simulink model "gm_stream_adaptation_model"  (R2020b)
settings: Solver=FixedStepDiscrete  StartTime=0.0  StopTime=2  RelTol=1e-3
undefined symbols (not defined in the file or in its folder): frame
libraries: hdlmdlgenlib x16, hdlsllib x2, simulink x2, whdlio x1
settings Model: Creator=wardo  LastModifiedBy=wardo
settings DataIOCC: LimitDataPoints=on  SaveOutput=off  SaveTime=off
settings OptimizationCC: BlockReduction=off  ConditionallyExecuteInputs=off  DefaultParameterBehavior=Inlined  LifeSpan=inf
settings DebuggingCC: AlgebraicLoopMsg=error  InheritedTsInSrcMsg=none  SingleTaskRateTransMsg=error  AllowSymbolicDim=off  StrictBusMsg=ErrorOnBusTreatedAsVector  SFUnexpectedBacktrackingDiag=warning  SFNoUnconditionalDefaultTransitionDiag=warning  SFExecutionAtInitializationDiag=none  ArithmeticOperatorsInVariantConditions=warning
settings HardwareCC: ProdBitPerPointer=32  ProdBitPerSizeT=32  ProdBitPerPtrDiffT=32  ProdLargestAtomicFloat=None  ProdIntDivRoundTo=Undefined  ProdEndianess=Unspecified  ProdWordSize=32  ProdHWDeviceType=ASIC/FPGA->ASIC/FPGA  ProdEqTarget=off
settings SFSimCC: SimUseLocalCustomCode=off  CustomCodeUndefinedFunction=UseInterfaceOnly
settings RTWCC: RTWUseLocalCustomCode=off
settings CodeAppCC: StateflowObjectComments=on
settings GRTTargetCC: TargetLangStandard=C89/C90 (ANSI)
settings ConfigComp: CovScope=ReferencedModels  CovMetricSettings=dw  CovSaveCumulativeToWorkspaceVar=on  CovSaveSingleToWorkspaceVar=on  CovExternalEMLEnable=off  CovSFcnEnable=off

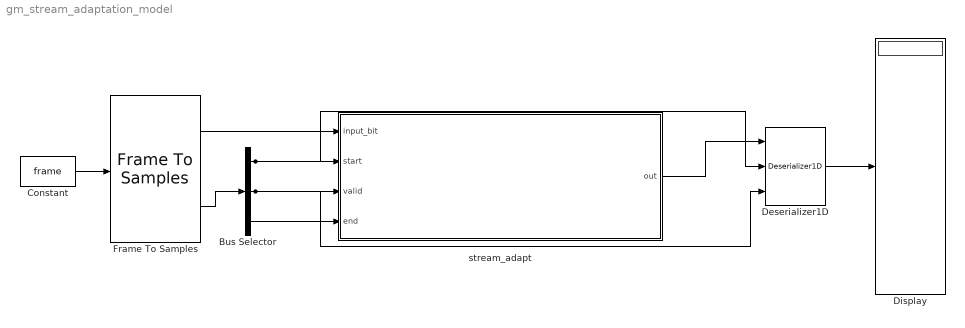
== system gm_stream_adaptation_model ==
  Bus Selector : BusSelector  OutputSignals=start,valid,end
  Constant : Constant  Value=frame  OutDataTypeStr=fixdt(1,16)  SampleTime=1
  Deserializer1D : hdlsllib/HDL Operations/Deserializer1D  Ratio=48408  IdleCycles=0  InitialCondition=0  startIn=on  validIn=on  validOut=off  inputDataDimensions=-1  inputSampleTime=-1  inputSignalType=auto
      settings: SourceProductBaseCode=SL
  Display : Display
  Frame To Samples : whdlio/Frame To Samples  InterSampleIdleCycles=0  InterFrameIdleCycles=0  OutputSize=1  InterleaveSamples=off
      settings: SourceProductBaseCode=LH
  stream_adapt : Subsystem
  wires:
  Deserializer1D/1 -> Display/1
  stream_adapt/1(out) -> Deserializer1D/1
  Bus Selector/3 -> stream_adapt/4(end)
  Bus Selector/2 -> stream_adapt/3(valid), Deserializer1D/3
  Bus Selector/1 -> stream_adapt/2(start), Deserializer1D/2
  Frame To Samples/2 -> Bus Selector/1
  Frame To Samples/1 -> stream_adapt/1(input_bit)
  Constant/1 -> Frame To Samples/1

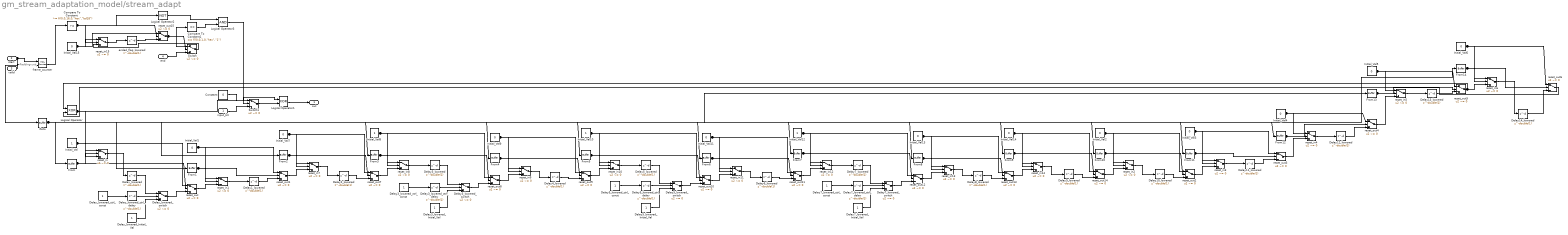
== system gm_stream_adaptation_model/stream_adapt ==
  note: Padding unit
  input_bit : Inport  OutDataTypeStr=fixdt(1, 16, 14)  PortDimensions=1  SampleTime=2.06577425218972e-05
  start : Inport  Port=2  OutDataTypeStr=boolean  PortDimensions=1  SampleTime=2.06577425218972e-05
  valid : Inport  Port=3  OutDataTypeStr=boolean  PortDimensions=1  SampleTime=2.06577425218972e-05
  end : Inport  Port=4  OutDataTypeStr=boolean  PortDimensions=1  SampleTime=2.06577425218972e-05
  Compare To Constant : simulink/Logic and Bit Operations/Compare To Constant  relop=>=  const="fi(0,0,16,0,\"hex\",\"bd18\")"  OutDataTypeStr=boolean
  Compare To Constant1 : simulink/Logic and Bit Operations/Compare To Constant  relop===  const="fi(0,0,1,0,\"hex\",\"1\")"  OutDataTypeStr=boolean
  Constant : Constant  Value=0  OutDataTypeStr=fixdt(0, 1, 1000)  SampleTime=2.06577425218972e-05
  Delay10_lowered : Delay  DelayLength=double(1)  InitialCondition=0  SampleTime=2.06577425218972e-05
  Delay11_lowered : Delay  DelayLength=double(1)  InitialCondition=0  SampleTime=2.06577425218972e-05
  Delay12_lowered : Delay  DelayLength=double(1)  InitialCondition=0  SampleTime=2.06577425218972e-05
  Delay13_lowered : Delay  DelayLength=double(1)  InitialCondition=0  SampleTime=2.06577425218972e-05
  Delay14_lowered : Delay  DelayLength=double(1)  InitialCondition=0  SampleTime=2.06577425218972e-05
  Delay1_lowered : Delay  DelayLength=double(1)  InitialCondition=0  SampleTime=2.06577425218972e-05
  Delay2_lowered : Delay  DelayLength=double(1)  InitialCondition=0  SampleTime=2.06577425218972e-05
  Delay3_lowered : Delay  DelayLength=double(1)  InitialCondition=0  SampleTime=2.06577425218972e-05
  Delay3_lowered_Initial_Val : Constant  OutDataTypeStr=boolean  SampleTime=2.06577425218972e-05
  Delay3_lowered_ctrl_const : Constant  OutDataTypeStr=boolean  SampleTime=2.06577425218972e-05
  Delay3_lowered_ctrl_delay : Delay  DelayLength=double(1)  InitialCondition=0  SampleTime=2.06577425218972e-05
  Delay3_lowered_switch : Switch  Criteria=u2 ~= 0  Threshold=double(0)  OutDataTypeStr=boolean  SampleTime=2.06577425218972e-05
  Delay4_lowered : Delay  DelayLength=double(1)  InitialCondition=0  SampleTime=2.06577425218972e-05
  Delay5_lowered : Delay  DelayLength=double(1)  InitialCondition=0  SampleTime=2.06577425218972e-05
  Delay5_lowered_Initial_Val : Constant  OutDataTypeStr=boolean  SampleTime=2.06577425218972e-05
  Delay5_lowered_ctrl_const : Constant  OutDataTypeStr=boolean  SampleTime=2.06577425218972e-05
  Delay5_lowered_ctrl_delay : Delay  DelayLength=double(1)  InitialCondition=0  SampleTime=2.06577425218972e-05
  Delay5_lowered_switch : Switch  Criteria=u2 ~= 0  Threshold=double(0)  OutDataTypeStr=boolean  SampleTime=2.06577425218972e-05
  Delay6_lowered : Delay  DelayLength=double(1)  InitialCondition=0  SampleTime=2.06577425218972e-05
  Delay7_lowered : Delay  DelayLength=double(1)  InitialCondition=0  SampleTime=2.06577425218972e-05
  Delay7_lowered_Initial_Val : Constant  OutDataTypeStr=boolean  SampleTime=2.06577425218972e-05
  Delay7_lowered_ctrl_const : Constant  OutDataTypeStr=boolean  SampleTime=2.06577425218972e-05
  Delay7_lowered_ctrl_delay : Delay  DelayLength=double(1)  InitialCondition=0  SampleTime=2.06577425218972e-05
  Delay7_lowered_switch : Switch  Criteria=u2 ~= 0  Threshold=double(0)  OutDataTypeStr=boolean  SampleTime=2.06577425218972e-05
  Delay8_lowered : Delay  DelayLength=double(1)  InitialCondition=0  SampleTime=2.06577425218972e-05
  Delay9_lowered : Delay  DelayLength=double(1)  InitialCondition=0  SampleTime=2.06577425218972e-05
  Delay_lowered : Delay  DelayLength=double(1)  InitialCondition=0  SampleTime=2.06577425218972e-05
  Delay_lowered_Initial_Val : Constant  OutDataTypeStr=boolean  SampleTime=2.06577425218972e-05
  Delay_lowered_ctrl_const : Constant  OutDataTypeStr=boolean  SampleTime=2.06577425218972e-05
  Delay_lowered_ctrl_delay : Delay  DelayLength=double(1)  InitialCondition=0  SampleTime=2.06577425218972e-05
  Delay_lowered_switch : Switch  Criteria=u2 ~= 0  Threshold=double(0)  OutDataTypeStr=boolean  SampleTime=2.06577425218972e-05
  From{,1..14} (15 alike) : hdlmdlgenlib/Buffer
      settings: SourceProductBaseCode=SL
  Goto : hdlmdlgenlib/Buffer
      settings: SourceProductBaseCode=SL
  Initial_Val{,8,10,12} (4 alike) : Constant  OutDataTypeStr=boolean  SampleTime=2.06577425218972e-05
  Initial_Val{1..7,9,11,13..15} (12 alike) : Constant  Value=0  OutDataTypeStr=boolean  SampleTime=2.06577425218972e-05
  Logical Operator : Logic  Operator=XOR  AllPortsSameDT=off  OutDataTypeStr=boolean  SampleTime=2.06577425218972e-05
  Logical Operator1 : Logic  Operator=XOR  AllPortsSameDT=off  OutDataTypeStr=boolean  SampleTime=2.06577425218972e-05
  Logical Operator2 : Logic  Operator=NOT  Inputs=1  AllPortsSameDT=off  OutDataTypeStr=boolean  SampleTime=2.06577425218972e-05
  Logical Operator3 : Logic  AllPortsSameDT=off  OutDataTypeStr=boolean  SampleTime=2.06577425218972e-05
  Switch : Switch  Criteria=u2 ~= 0  Threshold=double(0)  OutDataTypeStr=boolean  SampleTime=2.06577425218972e-05
  Switch1 : Switch  Criteria=u2 ~= 0  Threshold=double(0)  OutDataTypeStr=fixdt(1, 16, 14)  SampleTime=2.06577425218972e-05
  ended_flag_lowered : Delay  DelayLength=double(1)  InitialCondition=0  SampleTime=2.06577425218972e-05
  frame_counter : hdlsllib/Sources/HDL Counter  CountType=Count limited  CountInit=double(0)  CountStep=double(1)  CountMax=double(48408)  CountFromType=Initial value  CountFrom=double(0)  CountResetPort=on  CountLoadPort=off  CountEnbPort=on  CountDirPort=off  CountDataType=Unsigned  CountWordLen=16  CountFracLen=0  CountSampTime=2.06577425218972e-05
  reset_in{,1..15} (16 alike) : Switch  Criteria=u2 ~= 0  Threshold=double(0)  OutDataTypeStr=boolean  SampleTime=2.06577425218972e-05
  reset_out{,1..15} (16 alike) : Switch  Criteria=u2 ~= 0  Threshold=double(0)  OutDataTypeStr=boolean  SampleTime=2.06577425218972e-05
  out : Outport  VectorParamsAs1DForOutWhenUnconnected=off
  wires:
  input_bit/1 -> Switch1/3
  start/1 -> frame_counter/1, Goto/1
  valid/1 -> frame_counter/2
  end/1 -> Switch/3
  Compare To Constant/1 -> Logical Operator2/1, reset_out15/2, reset_in15/2
  Compare To Constant1/1 -> Logical Operator3/2
  Constant/1 -> Switch1/1
  reset_out/1 -> reset_in1/3
  reset_out1/1 -> reset_in7/3
  reset_out2/1 -> reset_in3/3
  reset_out3/1 -> reset_in4/3
  reset_out4/1 -> reset_in5/3
  reset_out5/1 -> Logical Operator/1, reset_in6/3
  reset_out6/1 -> Logical Operator/2
  reset_out7/1 -> reset_in8/3
  reset_out8/1 -> reset_in9/3
  reset_out9/1 -> reset_in10/3
  reset_out10/1 -> reset_in11/3
  reset_out11/1 -> reset_in12/3
  reset_out12/1 -> reset_in13/3
  reset_out13/1 -> reset_in14/3
  reset_out14/1 -> reset_in2/3
  From/1 -> reset_out/2, reset_in/2
  From1/1 -> reset_out1/2, reset_in1/2
  From10/1 -> reset_out2/2, reset_in2/2
  From11/1 -> reset_out3/2, reset_in3/2
  From12/1 -> reset_out4/2, reset_in4/2
  From13/1 -> reset_out5/2, reset_in5/2
  From14/1 -> reset_out6/2, reset_in6/2
  From2/1 -> reset_out7/2, reset_in7/2
  From3/1 -> reset_out8/2, reset_in8/2
  From4/1 -> reset_out9/2, reset_in9/2
  From5/1 -> reset_out10/2, reset_in10/2
  From6/1 -> reset_out11/2, reset_in11/2
  From7/1 -> reset_out12/2, reset_in12/2
  From8/1 -> reset_out13/2, reset_in13/2
  From9/1 -> reset_out14/2, reset_in14/2
  Logical Operator/1 -> Logical Operator1/1, reset_in/3
  Logical Operator1/1 -> out/1
  Logical Operator2/1 -> Logical Operator3/1
  Logical Operator3/1 -> Switch1/2
  Switch/1 -> reset_in15/3
  Switch1/1 -> Logical Operator1/2
  reset_out15/1 -> Switch/2, Switch/1, Compare To Constant1/1
  frame_counter/1 -> Compare To Constant/1
  Goto/1 -> From9/1, From8/1, From7/1, From6/1, From5/1, From4/1, From3/1, From2/1, From14/1, From13/1, From12/1, From11/1, From10/1, From1/1, From/1
  Initial_Val/1 -> reset_out/1, reset_in/1
  Delay_lowered_switch/1 -> reset_out/3
  reset_in/1 -> Delay_lowered/1
  Initial_Val1/1 -> reset_out1/1, reset_in1/1
  Delay1_lowered/1 -> reset_out1/3
  reset_in1/1 -> Delay1_lowered/1
  Initial_Val2/1 -> reset_out2/1, reset_in2/1
  Delay10_lowered/1 -> reset_out2/3
  reset_in2/1 -> Delay10_lowered/1
  Initial_Val3/1 -> reset_out3/1, reset_in3/1
  Delay11_lowered/1 -> reset_out3/3
  reset_in3/1 -> Delay11_lowered/1
  Initial_Val4/1 -> reset_out4/1, reset_in4/1
  Delay12_lowered/1 -> reset_out4/3
  reset_in4/1 -> Delay12_lowered/1
  Initial_Val5/1 -> reset_out5/1, reset_in5/1
  Delay13_lowered/1 -> reset_out5/3
  reset_in5/1 -> Delay13_lowered/1
  Initial_Val6/1 -> reset_out6/1, reset_in6/1
  Delay14_lowered/1 -> reset_out6/3
  reset_in6/1 -> Delay14_lowered/1
  Initial_Val7/1 -> reset_out7/1, reset_in7/1
  Delay2_lowered/1 -> reset_out7/3
  reset_in7/1 -> Delay2_lowered/1
  Initial_Val8/1 -> reset_out8/1, reset_in8/1
  Delay3_lowered_switch/1 -> reset_out8/3
  reset_in8/1 -> Delay3_lowered/1
  Initial_Val9/1 -> reset_out9/1, reset_in9/1
  Delay4_lowered/1 -> reset_out9/3
  reset_in9/1 -> Delay4_lowered/1
  Initial_Val10/1 -> reset_out10/1, reset_in10/1
  Delay5_lowered_switch/1 -> reset_out10/3
  reset_in10/1 -> Delay5_lowered/1
  Initial_Val11/1 -> reset_out11/1, reset_in11/1
  Delay6_lowered/1 -> reset_out11/3
  reset_in11/1 -> Delay6_lowered/1
  Initial_Val12/1 -> reset_out12/1, reset_in12/1
  Delay7_lowered_switch/1 -> reset_out12/3
  reset_in12/1 -> Delay7_lowered/1
  Initial_Val13/1 -> reset_out13/1, reset_in13/1
  Delay8_lowered/1 -> reset_out13/3
  reset_in13/1 -> Delay8_lowered/1
  Initial_Val14/1 -> reset_out14/1, reset_in14/1
  Delay9_lowered/1 -> reset_out14/3
  reset_in14/1 -> Delay9_lowered/1
  Initial_Val15/1 -> reset_out15/1, reset_in15/1
  ended_flag_lowered/1 -> reset_out15/3
  reset_in15/1 -> ended_flag_lowered/1
  Delay_lowered/1 -> Delay_lowered_switch/1
  Delay_lowered_Initial_Val/1 -> Delay_lowered_switch/3
  Delay_lowered_ctrl_const/1 -> Delay_lowered_ctrl_delay/1
  Delay_lowered_ctrl_delay/1 -> Delay_lowered_switch/2
  Delay3_lowered/1 -> Delay3_lowered_switch/1
  Delay3_lowered_Initial_Val/1 -> Delay3_lowered_switch/3
  Delay3_lowered_ctrl_const/1 -> Delay3_lowered_ctrl_delay/1
  Delay3_lowered_ctrl_delay/1 -> Delay3_lowered_switch/2
  Delay5_lowered/1 -> Delay5_lowered_switch/1
  Delay5_lowered_Initial_Val/1 -> Delay5_lowered_switch/3
  Delay5_lowered_ctrl_const/1 -> Delay5_lowered_ctrl_delay/1
  Delay5_lowered_ctrl_delay/1 -> Delay5_lowered_switch/2
  Delay7_lowered/1 -> Delay7_lowered_switch/1
  Delay7_lowered_Initial_Val/1 -> Delay7_lowered_switch/3
  Delay7_lowered_ctrl_const/1 -> Delay7_lowered_ctrl_delay/1
  Delay7_lowered_ctrl_delay/1 -> Delay7_lowered_switch/2
